simulink model "sldemo_bounce_mod"  (R2025b)
settings: Solver=ode23  StartTime=0.0  StopTime=25  MaxStep=0.01  RelTol=1e-3  AbsTol=1E-6  EnableMultiTasking=on
undefined symbols (not defined in the file): g_acc, init_vel, k_rest
Description:
  | Bouncing Ball Model
  | 
  | This model calculates the trajectory, over time, of a ball thrown
  | upward with a velocity of 15 meters per second from a height of 10 m.
  | The model demonstrates the use of the 'ReinitDXDTwhenXreachesSaturation'
  | parameter in the Second-Order Integrator block to model this system.
  | This parameter, when set to 'on', forces a reinitialization of dx/dt
  | (velocity in the model) at the instant when x (position) reaches
  | saturation (i.e., when the ball hits the ground). The reinitialized value
  | is calculated by multiplying a coefficient of restitution times the ball
  | velocity, the instant before the ball hits the ground. The Memory block
  | in the calculation loop serves to capture the velocity of the ball just
  | before it hits the ground. The position of the ball is plotted in the
  | upper axis of the scope while the velocity of the ball is plotted in
  | the lower axis.
settings Model: ModifiedByFormat=The MathWorks, Inc.  Creator=The MathWorks, Inc.  LastModifiedBy=The MathWorks, Inc.
settings SolverCC: AutoScaleAbsTol=off  AlgebraicLoopSolver=TrustRegion
settings DataIOCC: MaxDataPoints=7500  DSMLogging=off  SaveTime=off  ReturnWorkspaceOutputs=off
settings OptimizationCC: ReuseModelBlockBuffer=off  ExpressionDepthLimit=2147483647.0  EfficientFloat2IntCast=on  LifeSpan=inf
settings DebuggingCC: UnderspecifiedInitializationDetection=Classic  MergeDetectMultiDrivingBlocksExec=none  IgnoredZcDiagnostic=none  FcnCallInpInsideContextMsg=warning  UnconnectedInputMsg=warning  UnconnectedOutputMsg=warning  UnconnectedLineMsg=warning  StateNameClashWarn=warning  SFUnexpectedBacktrackingDiag=warning  SFNoUnconditionalDefaultTransitionDiag=warning  SFExecutionAtInitializationDiag=none  ArithmeticOperatorsInVariantConditions=warning
settings HardwareCC: ProdBitPerPointer=32.0  ProdBitPerSizeT=32.0  ProdBitPerPtrDiffT=32.0  ProdLargestAtomicFloat=None  ProdIntDivRoundTo=Undefined  ProdEndianess=Unspecified  ProdWordSize=32.0  ProdHWDeviceType=32-bit Generic  TargetBitPerLong=64.0  TargetBitPerPointer=64.0  TargetBitPerSizeT=64.0  TargetBitPerPtrDiffT=64.0  TargetLongLongMode=on  TargetIntDivRoundTo=Zero  TargetEndianess=LittleEndian  TargetWordSize=64.0  TargetHWDeviceType=MATLAB Host  ProdEqTarget=off
settings ModelReferenceCC: EnableRefExpFcnMdlSchedulingChecks=on  PropagateSignalLabelsOutOfModel=off
settings SFSimCC: SimUseLocalCustomCode=off  CustomCodeUndefinedFunction=UseInterfaceOnly
settings RTWCC: SystemTargetFile=rsim.tlc  TemplateMakefile=rsim_default_tmf  RTWUseLocalCustomCode=off  GPUComputeCapability=3.5  Description=Rapid Simulation Target
settings CodeAppCC: StateflowObjectComments=on
settings RSimTargetCC: ExtModeTransport=0.0  ExtModeStaticAllocSize=1000000.0  TargetLangStandard=C99 (ISO)  MultiwordLength=2048.0  DynamicStringBufferSize=256.0  PreserveMATLABNamespacesInGeneratedCode=on  SubcomponentCodeInterfacePackaging=Reusable function  InstructionSetFMA=off  OptimizeReductions=off  LogToMDFFile=off
settings ConfigComp: CovMetricSettings=dw  CovSaveCumulativeToWorkspaceVar=on  CovSaveSingleToWorkspaceVar=on  CovExternalEMLEnable=off

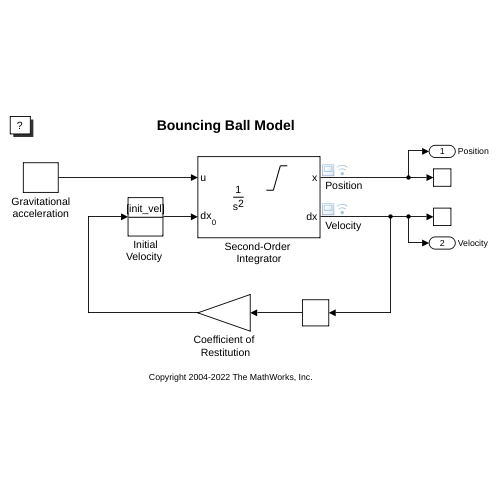
[thumbnail: Simulink's stored preview of the top-level diagram]
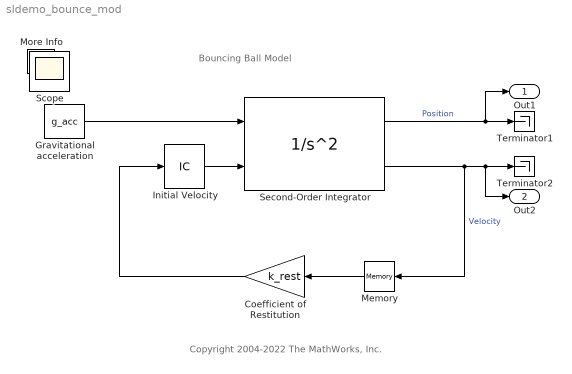
== system sldemo_bounce_mod ==
  note: Bouncing Ball Model
  note: Copyright 2004-2022 The MathWorks, Inc.
  Coefficient of Restitution : Gain  Gain=k_rest
  Gravitational acceleration : Constant  Value=g_acc  OutDataTypeStr=double
  "Initial Velocity " : InitialCondition  Value=init_vel
  Memory : Memory
  More Info : Subsystem
      settings: OpenFcn=showExample('simulink_general/sldemo_bounceExample')
      mask Display: disp('?')
  Second-Order Integrator : SecondOrderIntegrator  ICX=init_pos  LimitX=on  LowerLimitX=0.0  StateNameX='Position'  ICSourceDXDT=external  StateNameDXDT='Velocity'  ReinitDXDTwhenXreachesSaturation=on
  Terminator1 : Terminator
  Terminator2 : Terminator
  Out1 : Outport  SignalName=Position
  Out2 : Outport  Port=2  SignalName=Velocity
  Scope : Scope
      settings: ActiveDisplayYMinimum=0  ActiveDisplayYMaximum=25  DataLoggingMaxPoints=7500  DataLoggingSaveFormat=Array
  wires:
  Gravitational acceleration/1 -> Second-Order Integrator/1
  Second-Order Integrator/1 -> Out1/1, Terminator1/1  "Position"
  Second-Order Integrator/2 -> Memory/1, Out2/1, Terminator2/1  "Velocity"
  Memory/1 -> Coefficient of Restitution/1
  "Initial Velocity "/1 -> Second-Order Integrator/2
  Coefficient of Restitution/1 -> "Initial Velocity "/1

== system sldemo_bounce_mod/More Info ==
